simulink library "fdclib4"  (Simulink 3.00)
undefined symbols (not defined in the file): GM1
settings Model: LastModifiedBy=Dutchroll

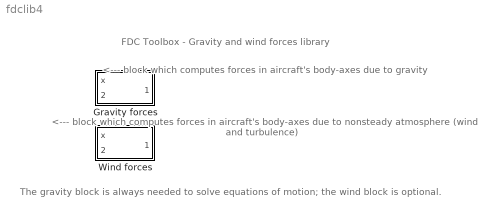
== system fdclib4 ==
  note: FDC Toolbox - Gravity and wind forces library
  note: The gravity block is always needed to solve
      | equations of motion; the wind block is optional.
  note: <--- block which computes forces in
      | aircraft's body-axes due to gravity
  note: <--- block which computes forces in
      | aircraft's body-axes due to nonsteady
      | atmosphere (wind and turbulence)
  Gravity forces : Subsystem  mask(Gravity){m=GM1(10)}
      mask prompts: m "Mass of the aircraft [kg]:"
      mask help: Gravity forces.
      mask Help: eval('browse gravity')
      mask Display: disp('Gravity')
  Wind forces : Subsystem  mask(fwind){m=GM1(10)}
      mask prompts: m "Mass of the aircraft [kg]:"
      mask help: Forces due to non-steady atmosphere.
      mask Help: eval('browse fwind')
      mask Display: disp('Fwind')

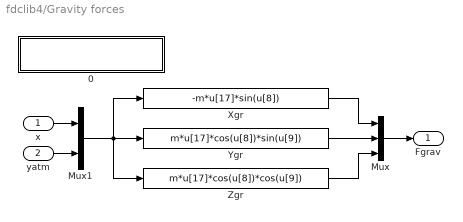
== system fdclib4/Gravity forces ==
  x : Inport  Port=1  PortWidth=-1  SampleTime=-1  DataType=auto
      settings: SignalType=auto
  yatm : Inport  Port=2  PortWidth=-1  SampleTime=-1  DataType=auto
      settings: SignalType=auto
  0 : Subsystem
      settings: OpenFcn=browse gravity
      mask Display: disp('GRAVITY\nM.O. Rauw, March 2003')
  Mux : Mux  Inputs=3
      settings: DisplayOption=none
  Mux1 : Mux  Inputs=[12 5]
      settings: DisplayOption=none
  Xgr : Fcn  Expr=-m*u[17]*sin(u[8])
  Ygr : Fcn  Expr=m*u[17]*cos(u[8])*sin(u[9])
  Zgr : Fcn  Expr=m*u[17]*cos(u[8])*cos(u[9])
  Fgrav : Outport  Port=1
  wires:
  yatm/1 -> Mux1/2
  x/1 -> Mux1/1
  Zgr/1 -> Mux/3
  Mux1/1 -> Zgr/1, Xgr/1, Ygr/1
  Mux/1 -> Fgrav/1
  Ygr/1 -> Mux/2
  Xgr/1 -> Mux/1

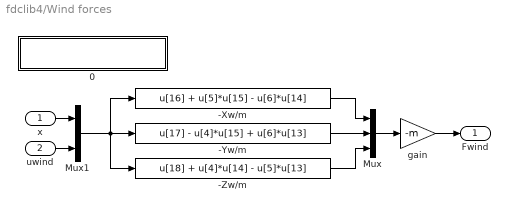
== system fdclib4/Wind forces ==
  x : Inport  Port=1  PortWidth=-1  SampleTime=-1  DataType=auto
      settings: SignalType=auto
  uwind : Inport  Port=2  PortWidth=-1  SampleTime=-1  DataType=auto
      settings: SignalType=auto
  -Xw/m : Fcn  Expr=u[16] + u[5]*u[15] - u[6]*u[14]
  -Yw/m : Fcn  Expr=u[17] - u[4]*u[15] + u[6]*u[13]
  -Zw/m : Fcn  Expr=u[18] + u[4]*u[14] - u[5]*u[13]
  0 : Subsystem
      settings: OpenFcn=browse fwind
      mask Display: disp('FWIND\nM.O. Rauw, March 2003')
  Mux : Mux  Inputs=3
      settings: DisplayOption=none
  Mux1 : Mux  Inputs=[12 6]
      settings: DisplayOption=none
  gain : Gain  Gain=-m  SaturateOnIntegerOverflow=on
  Fwind : Outport  Port=1
  wires:
  -Zw/m/1 -> Mux/3
  -Xw/m/1 -> Mux/1
  -Yw/m/1 -> Mux/2
  Mux1/1 -> -Xw/m/1, -Zw/m/1, -Yw/m/1
  Mux/1 -> gain/1
  x/1 -> Mux1/1
  uwind/1 -> Mux1/2
  gain/1 -> Fwind/1

== system fdclib4/Gravity forces/0 ==

== system fdclib4/Wind forces/0 ==
